simulink model "AccTarSel"  (R2018b)
settings: Solver=FixedStepDiscrete  StartTime=0.0  StopTime=inf  FixedStep=0.01  RelTol=1e-3
PostLoadFcn:
  | if any(exist('dsrtsu_mdlpostloadfcn', 'file') ~= 0), dsrtsu_mdlpostloadfcn('Execute', bdroot); end
values from neighbouring files (symbols this model uses):
  P_adtMaxBDC = 1.0    [AccTarSel.sldd]
  P_aFOCApproachIntpAcitve = -0.6    [AccTarSel.sldd]
  P_aFOCApproachIntpEnsure = -1.8    [AccTarSel.sldd]
  P_CutInEnable = 1.0    [AccTarSel.sldd]
  P_dAimMin = 4.5    [AccTarSel.sldd]
  P_dAimMinAVP = 1.5    [AccTarSel.sldd]
  P_dObjDrvOffMax = 5.0    [AccTarSel.sldd]
  P_dObjDrvOffMin = 3.0    [AccTarSel.sldd]
  P_dObjLowHystDecToStop = 4.5    [AccTarSel.sldd]
  P_dObjLowHystDecToStopAVP = 1.5    [AccTarSel.sldd]
  P_dObjUpperHystDecToStop = 5.0    [AccTarSel.sldd]
  P_dResMax = 5.0    [AccTarSel.sldd]
  P_dStandStill = 3.0    [AccTarSel.sldd]
  P_dStandStillMin = 2.0    [AccTarSel.sldd]
  P_dvarYMax4PO = 1.0    [AccTarSel.sldd]
  P_dyCutInThres = 3.6    [AccTarSel.sldd]
  P_facBDCInit = 0.7    [AccTarSel.sldd]
  P_facBDCIterCalc = 0.8    [AccTarSel.sldd]
  P_facFOCNegDiff = 0.3    [AccTarSel.sldd]
  P_facFOCPosDiff = 0.2    [AccTarSel.sldd]
  P_kapHystThres = 0.0005    [AccTarSel.sldd]
  P_PlausIntegDisable = 0.0    [AccTarSel.sldd]
  P_plausMin4PO = 0.5    [AccTarSel.sldd]
  P_probExistMin4PO = 0.8    [AccTarSel.sldd]
  P_StandObjEnable = 0.0    [AccTarSel.sldd]
  P_tAxTrackNegLower = 0.3    [AccTarSel.sldd]
  P_tAxTrackNegUpper = 0.6    [AccTarSel.sldd]
  P_tAxTrackPosLower = 1.0    [AccTarSel.sldd]
  P_tAxTrackPosUpper = 2.0    [AccTarSel.sldd]
  P_tBDCStartFilt = 0.2    [AccTarSel.sldd]
  P_tCSC = 3.5    [AccTarSel.sldd]
  P_tCurvFilt = 0.2    [AccTarSel.sldd]
  P_tCutInFilt = 0.5    [AccTarSel.sldd]
  P_tFiltAxAbsPONegFast = 0.1    [AccTarSel.sldd]
  P_tFiltAxAbsPONegSlow = 0.4    [AccTarSel.sldd]
  P_tFiltAxAbsPOPosFast = 1.2    [AccTarSel.sldd]
  P_tFiltAxAbsPOPosSlow = 2.0    [AccTarSel.sldd]
  P_tFiltAxAbsPOStand = 2.0    [AccTarSel.sldd]
  P_tFiltDAim = 0.1    [AccTarSel.sldd]
  P_tFiltDsd = 0.1    [AccTarSel.sldd]
  P_tFiltSpdLim = 3.0    [AccTarSel.sldd]
  P_tFiltVxAxPOFast = 0.15    [AccTarSel.sldd]
  P_tFiltVxAxPOSlow = 0.25    [AccTarSel.sldd]
  P_tFOCStatAccelFast = 4.0    [AccTarSel.sldd]
  P_tFOCStatAccelSlow = 3.5    [AccTarSel.sldd]
  P_tFOCStatDecelFast = 4.0    [AccTarSel.sldd]
  P_tFOCStatDecelSlow = 3.2    [AccTarSel.sldd]
  P_tMinDrvPhase = 2.0    [AccTarSel.sldd]
  P_tPredObjLeav = 1.2    [AccTarSel.sldd]
  P_tRollingFilt = 0.5    [AccTarSel.sldd]
  P_tRollingFinFilt = 1.0    [AccTarSel.sldd]
  P_tSSCNeg = 4.5    [AccTarSel.sldd]
  P_tSSCPos = 5.5    [AccTarSel.sldd]
  P_tToStop = 5.0    [AccTarSel.sldd]
  P_tToStopInBDC = 6.0    [AccTarSel.sldd]
  P_tToStopTrig = 4.0    [AccTarSel.sldd]
  P_vEgoDecToStop = 3.0    [AccTarSel.sldd]
  P_vEgoLowBDC = 4.0    [AccTarSel.sldd]
  P_vFOCNegDiff = 4.0    [AccTarSel.sldd]
  P_vFOCPosDiff = 5.0    [AccTarSel.sldd]
  P_vFOCStationaryFast = 15.0    [AccTarSel.sldd]
  P_vFOCStationarySlow = 5.0    [AccTarSel.sldd]
  P_vObjDrvOff = 0.5    [AccTarSel.sldd]
  P_vObjLowHystDecToStop = 0.5    [AccTarSel.sldd]
  P_vObjNoStop = 1.0    [AccTarSel.sldd]
  P_vObjReCalc = 1.0    [AccTarSel.sldd]
  P_vObjStop = 0.3    [AccTarSel.sldd]
  P_vObjUpperHystDecToStop = 0.8    [AccTarSel.sldd]
  P_vStandStill = 0.3    [AccTarSel.sldd]
  P_vStandStillHyst = 0.3    [AccTarSel.sldd]
  P_vyCutInThres = 0.5    [AccTarSel.sldd]
libraries: simulink x21, LPFilter x12
(part 11 of 11)

== system AccTarSel/ACC_Control/FollowObjCtrl/FollowObjValid/BrakeDistCtrl/calcA/If Action Subsystem/If Action Subsystem1 ==
  t : Inport
  aMax : Inport  Port=2
  adt2 : Inport  Port=3
  T30 : Inport  Port=4
  dRes : Inport  Port=5
  aCharactK1 : Inport  Port=6
  SYS_Info_st : Inport  Port=7
  Action Port : ActionPort  ActionType=elseif
  Add : Sum
  Add1 : Sum  Inputs=+-
  Bus Selector : BusSelector  OutputSignals=dT
  Constant : Constant
  Constant2 : Constant  Value=0  OutDataTypeStr=single
  LPFilter : LPFilter/LPFilter  SystemSampleTime=-1
      settings: SourceProductName=CustomLib
  LPFilter1 : LPFilter/LPFilter  SystemSampleTime=-1
      settings: SourceProductName=CustomLib
  Multiply : Product
  P_tRollingFilt : Constant  Value=P_tRollingFilt  OutDataTypeStr=single
  P_tRollingFinFilt : Constant  Value=P_tRollingFinFilt  OutDataTypeStr=single
  Relational Operator : RelationalOperator  Operator=>  OutDataTypeStr=boolean  RndMeth=Simplest
  Switch : Switch  Criteria=u2 > Threshold
  Out1 : Outport
  wires:
  aMax/1 -> Add/1
  t/1 -> Add1/1
  T30/1 -> Add1/2
  Add1/1 -> Multiply/1
  adt2/1 -> Multiply/2
  Multiply/1 -> Add/2
  Constant/1 -> Relational Operator/2
  dRes/1 -> Relational Operator/1
  Relational Operator/1 -> Switch/2
  Switch/1 -> Out1/1
  aCharactK1/1 -> LPFilter/4, LPFilter1/4
  SYS_Info_st/1 -> Bus Selector/1
  Bus Selector/1 -> LPFilter/2, LPFilter1/2  "<dT>"
  LPFilter/1 -> Switch/1
  P_tRollingFilt/1 -> LPFilter/3
  Constant2/1 -> LPFilter/1
  Add/1 -> LPFilter1/1
  P_tRollingFinFilt/1 -> LPFilter1/3
  LPFilter1/1 -> Switch/3

== system AccTarSel/ACC_Control/FollowObjCtrl/FollowObjValid/BrakeDistCtrl/calcA/If Action Subsystem/If Action Subsystem2 ==
  Action Port : ActionPort  ActionType=else
  Constant : Constant  Value=0  OutDataTypeStr=single
  Out1 : Outport
  wires:
  Constant/1 -> Out1/1

== system AccTarSel/ACC_Control/FollowObjCtrl/FollowObjValid/BrakeDistCtrl/calcA/If Action Subsystem/If Action Subsystem3 ==
  In1 : Inport
  Action Port : ActionPort  ActionType=then
  Out1 : Outport
  wires:
  In1/1 -> Out1/1

== system AccTarSel/ACC_Control/FollowObjCtrl/FollowObjValid/BrakeDistCtrl/calcA/If Action Subsystem/Subsystem ==
  aCharact : Inport
  a0Raw : Inport  Port=2
  tElapse : Inport  Port=3
  SYS_Info_st : Inport  Port=4
  aBDCK1 : Inport  Port=5
  Action Port : ActionPort  ActionType=else
  Bus Selector : BusSelector  OutputSignals=dT
  LPFilter : LPFilter/LPFilter  SystemSampleTime=-1
      settings: SourceProductName=CustomLib
  P_adtMaxBDC : Constant  Value=P_adtMaxBDC
  P_tBDCStartFilt : Constant  Value=P_tBDCStartFilt  OutDataTypeStr=single
  Relational Operator : RelationalOperator  Operator=<=  OutDataTypeStr=boolean  RndMeth=Simplest
  Switch : Switch  Criteria=u2 > Threshold
  Terminator : Terminator
  Out1 : Outport
  wires:
  tElapse/1 -> Relational Operator/1
  P_adtMaxBDC/1 -> Terminator/1
  a0Raw/1 -> Switch/1
  Bus Selector/1 -> LPFilter/2, Relational Operator/2  "<dT>"
  Relational Operator/1 -> Switch/2
  Switch/1 -> Out1/1
  SYS_Info_st/1 -> Bus Selector/1
  aBDCK1/1 -> LPFilter/4
  P_tBDCStartFilt/1 -> LPFilter/3
  aCharact/1 -> LPFilter/1
  LPFilter/1 -> Switch/3

== system AccTarSel/ACC_Control/FollowObjCtrl/FollowObjValid/BrakeDistCtrl/calcCriteria/calcObjStop/ObjNoStop ==
  Action Port : ActionPort  ActionType=then
  Constant2 : Constant  Value=255  OutDataTypeStr=single
  tToStop : Outport
  dToStop : Outport  Port=2
  wires:
  Constant2/1 -> dToStop/1, tToStop/1

== system AccTarSel/ACC_Control/FollowObjCtrl/FollowObjValid/BrakeDistCtrl/calcCriteria/calcObjStop/ObjStopped ==
  Action Port : ActionPort  ActionType=elseif
  Constant2 : Constant  Value=0  OutDataTypeStr=single
  tToStop : Outport
  dToStop : Outport  Port=2
  wires:
  Constant2/1 -> tToStop/1, dToStop/1

== system AccTarSel/ACC_Control/FollowObjCtrl/FollowObjValid/BrakeDistCtrl/calcCriteria/calcObjStop/ObjStopping ==
  vAbsObj : Inport
  aAbsObj : Inport  Port=2
  Action Port : ActionPort  ActionType=else
  Abs : Abs
  Abs1 : Abs
  Constant1 : Constant  Value=-0.1  OutDataTypeStr=single
  Constant2 : Constant  Value=2  OutDataTypeStr=single
  Divide1 : Product  Inputs=*/
  Divide2 : Product  Inputs=*/
  Min : MinMax  Inputs=2
  Multiply : Product
  Square : Math  Operator=square  SaturateOnIntegerOverflow=on
  tToStop : Outport
  dToStop : Outport  Port=2
  wires:
  vAbsObj/1 -> Square/1, Divide1/1
  Divide1/1 -> Abs/1
  Square/1 -> Divide2/1
  Constant2/1 -> Multiply/2
  Multiply/1 -> Divide2/2
  Divide2/1 -> Abs1/1
  Abs/1 -> tToStop/1
  Abs1/1 -> dToStop/1
  aAbsObj/1 -> Min/1
  Constant1/1 -> Min/2
  Min/1 -> Multiply/1, Divide1/2

== system AccTarSel/ACC_Control/FollowObjCtrl/FollowObjValid/BrakeDistCtrl/calcCriteria/calcObjStop/Subsystem ==
  StateK1 : Inport
  Constant2 : Constant  Value=3  OutDataTypeStr=single
  Constant3 : Constant  Value=2  OutDataTypeStr=single
  OR : Logic  Operator=OR  AllPortsSameDT=off  OutDataTypeStr=boolean
  P_tToStop : Constant  Value=P_tToStop  OutDataTypeStr=single
  P_tToStopInBDC : Constant  Value=P_tToStopInBDC  OutDataTypeStr=single
  Relational Operator : RelationalOperator  Operator===  OutDataTypeStr=boolean  RndMeth=Simplest
  Relational Operator1 : RelationalOperator  Operator===  OutDataTypeStr=boolean  RndMeth=Simplest
  Switch : Switch  Criteria=u2 > Threshold
  tStop : Outport
  wires:
  Relational Operator1/1 -> OR/2
  Relational Operator/1 -> OR/1
  OR/1 -> Switch/2
  Constant2/1 -> Relational Operator1/2
  StateK1/1 -> Relational Operator1/1, Relational Operator/1
  Constant3/1 -> Relational Operator/2
  P_tToStopInBDC/1 -> Switch/1
  P_tToStop/1 -> Switch/3
  Switch/1 -> tStop/1

== system AccTarSel/ACC_Control/FollowObjCtrl/FollowObjValid/BrakeDistCtrl/calcProfile/calc/Subsystem ==
  initCond : Inport
  Add : Sum  Inputs=+-
  Add1 : Sum  Inputs=+-
  Bus Creator : BusCreator  Inputs=8
  Bus Selector : BusSelector  OutputSignals=SmoothStopCond,a0,a0Raw
  Divide : Product  Inputs=*/
  Divide1 : Product  Inputs=*/
  Gain : Gain  Gain=-1
  Iteration : Subsystem  TreatAsAtomicUnit=on
  Profile : Outport
  wires:
  initCond/1 -> Iteration/1(initCond), Bus Selector/1
  Iteration/1(aMax) -> Bus Creator/2, Add/1, Gain/1
  Bus Selector/2 -> Bus Creator/7, Add/2  "<a0>"
  Add/1 -> Divide/1
  Iteration/3(T30) -> Bus Creator/4, Add1/2, Divide/2
  Divide/1 -> Bus Creator/5  "adt1"
  Iteration/2(T) -> Bus Creator/3, Add1/1
  Gain/1 -> Divide1/1
  Add1/1 -> Divide1/2
  Divide1/1 -> Bus Creator/6  "adt2"
  Bus Selector/1 -> Bus Creator/1  "<SmoothStopCond>"
  Bus Creator/1 -> Profile/1  "Profile"
  Bus Selector/3 -> Bus Creator/8  "<a0Raw>"

== system AccTarSel/ACC_Control/FollowObjCtrl/FollowObjValid/BrakeDistCtrl/calcProfile/calc/calcInitCondition ==
  note: a0 should be calculated by both aRef and last aCmd value
  egoInfo : Inport
  objInfo : Inport  Port=2
  dObjToStop : Inport  Port=3
  aCvK1 : Inport  Port=4
  Add : Sum  Inputs=++-
  Add1 : Sum
  Bus Selector : BusSelector  OutputSignals=aRef,vRef
  Bus Selector1 : BusSelector  OutputSignals=dx
  Constant : Constant  Value=-0.1  OutDataTypeStr=single
  Divide : Product  Inputs=*/
  Gain : Gain  Gain=-2/3
  Gain1 : Gain
  Gain2 : Gain  Gain=0.0
  Max : MinMax  Function=max  Inputs=2
  Min : MinMax  Inputs=2
  Multiply : Product
  Multiply1 : Product
  P_dStandStill : Constant  Value=P_dStandStill  OutDataTypeStr=single
  P_dStandStillMin : Constant  Value=P_dStandStillMin  OutDataTypeStr=single
  P_facBDCInit : Constant  Value=P_facBDCInit  OutDataTypeStr=single
  Square : Math  Operator=square  SaturateOnIntegerOverflow=on
  a0 : Outport
  aThres : Outport  Port=2
  v0 : Outport  Port=3
  v30 : Outport  Port=4
  dAimBDC : Outport  Port=5
  d30 : Outport  Port=6
  wires:
  egoInfo/1 -> Bus Selector/1
  Bus Selector/2 -> Multiply/1, v0/1, Square/1  "<vRef>"
  objInfo/1 -> Bus Selector1/1
  dObjToStop/1 -> Add/2
  Bus Selector1/1 -> Add/1  "<dx>"
  P_dStandStill/1 -> Add/3
  Add/1 -> Max/1
  P_dStandStillMin/1 -> Max/2
  Max/1 -> Divide/2, Multiply1/1, dAimBDC/1  "dAimBDC"
  Square/1 -> Divide/1
  Divide/1 -> Gain/1
  Gain/1 -> aThres/1
  Multiply/1 -> v30/1
  P_facBDCInit/1 -> Multiply1/2, Multiply/2
  Multiply1/1 -> d30/1
  aCvK1/1 -> Gain1/1
  Bus Selector/1 -> Gain2/1  "<aRef>"
  Gain1/1 -> Add1/1
  Gain2/1 -> Add1/2
  Add1/1 -> Min/2
  Constant/1 -> Min/1
  Min/1 -> a0/1

== system AccTarSel/ACC_Target_Selection/Subsystem/ValidObjCalc/CutInCalc/Subsystem/Subsystem/If Action Subsystem ==
  dy : Inport
  vy : Inport  Port=2
  Action Port : ActionPort  ActionType=then
  1-D Lookup Table : Lookup_n-D  NumberOfTableDimensions=1  LookupTableObject=''  BreakpointsForDimension1=[0.5,1.5]  BreakpointsForDimension1FirstPoint=10  BreakpointsForDimension2FirstPoint=10  BreakpointsForDimension1Spacing=12  BreakpointsForDimension2Spacing=12  IndexSearchMethod=Linear search  Table=[0,1.5]  ExtrapMethod=Clip  InternalRulePriority=Speed  RndMeth=Simplest  InputSameDT=on
  1-D Lookup Table1 : Lookup_n-D  NumberOfTableDimensions=1  LookupTableObject=''  BreakpointsForDimension1=[1,1.8]  BreakpointsForDimension1FirstPoint=10  BreakpointsForDimension2FirstPoint=10  BreakpointsForDimension1Spacing=12  BreakpointsForDimension2Spacing=12  IndexSearchMethod=Linear search  Table=[1,0]  ExtrapMethod=Clip  InternalRulePriority=Speed  RndMeth=Simplest  InputSameDT=on
  Abs : Abs
  Abs1 : Abs
  Add : Sum
  Constant : Constant  Value=0  OutDataTypeStr=single
  Max : MinMax  Function=max  Inputs=2
  Max1 : MinMax  Inputs=2
  Multiply : Product
  Switch : Switch  Criteria=u2 > Threshold
  Out1 : Outport
  Out2 : Outport  Port=2
  wires:
  vy/1 -> Multiply/1, Abs1/1
  1-D Lookup Table/1 -> Multiply/2  "tPred"
  dy/1 -> Switch/2, Add/1
  Multiply/1 -> Add/2
  Add/1 -> Max1/2, Max/1
  Constant/1 -> Max1/1, Max/2
  Switch/1 -> Out2/1, Abs/1  "dyPred"
  1-D Lookup Table1/1 -> Out1/1
  Abs/1 -> 1-D Lookup Table1/1
  Abs1/1 -> 1-D Lookup Table/1
  Max/1 -> Switch/1
  Max1/1 -> Switch/3

== system AccTarSel/ACC_Target_Selection/Subsystem/ValidObjCalc/CutInCalc/Subsystem/Subsystem/If Action Subsystem1 ==
  dy : Inport
  Action Port : ActionPort  ActionType=else
  Constant : Constant  Value=0  OutDataTypeStr=single
  Out1 : Outport
  Out2 : Outport  Port=2
  wires:
  Constant/1 -> Out1/1
  dy/1 -> Out2/1

== system AccTarSel/ACC_Control/FollowObjCtrl/FollowObjValid/BrakeDistCtrl/calcProfile/calc/Subsystem/Iteration ==
  initCond : Inport
  Add : Sum  Inputs=+-
  Add1 : Sum
  Add2 : Sum
  Add3 : Sum  Inputs=+++
  Bus Selector : BusSelector  OutputSignals=dAimBDC,d30,v30,a0,v0
  Constant : Constant  OutDataTypeStr=int32
  Divide : Product  Inputs=*/
  Divide1 : Product  Inputs=*/
  For Iterator : ForIterator  IterationLimit=10
  Gain : Gain  Gain=0.7
  Gain1 : Gain  Gain=3
  Gain2 : Gain  Gain=0.7
  Gain3 : Gain  Gain=-2
  Gain4 : Gain  Gain=0.3
  Gain5 : Gain  Gain=0.5
  Gain6 : Gain  Gain=1/3
  Gain7 : Gain  Gain=1/6
  Gain8 : Gain  Gain=0.3
  Memory{,1..3} (4 alike) : Memory  InheritSampleTime=on
  Multiply{,1..3} (4 alike) : Product
  Relational Operator : RelationalOperator  Operator===  OutDataTypeStr=boolean  RndMeth=Simplest
  Square : Math  Operator=square  SaturateOnIntegerOverflow=on
  calcD30 : Subsystem
  calcV30 : Subsystem
  aMax : Outport
  T : Outport  Port=2
  T30 : Outport  Port=3
  wires:
  initCond/1 -> Bus Selector/1
  Bus Selector/1 -> Add/1  "<dAimBDC>"
  calcD30/1(d30) -> Add/2, Memory2/1  "d30"
  calcV30/1(v30) -> Memory3/1, Gain/1, Gain3/1  "v30"
  Add/1 -> Divide/1
  Gain/1 -> Divide/2
  Divide/1 -> Gain1/1
  Gain1/1 -> Gain8/1, T/1, Gain4/1, Gain2/1  "T"
  Gain3/1 -> Divide1/1
  Gain2/1 -> Divide1/2  "0.7T"
  Divide1/1 -> aMax/1, Multiply3/1, Add2/1  "aMax"
  Gain4/1 -> Multiply1/1, Square/1, Multiply/2  "0.3T"
  Bus Selector/4 -> Multiply2/1, Add2/2  "<a0>"
  Multiply/1 -> Gain5/1
  Gain5/1 -> Add1/1
  Bus Selector/5 -> Multiply1/2, Add1/2  "<v0>"
  Add2/1 -> Multiply/1
  Add1/1 -> Memory1/1  "v30new"
  Square/1 -> Multiply3/2, Multiply2/2
  Multiply2/1 -> Gain6/1
  Multiply3/1 -> Gain7/1
  Gain6/1 -> Add3/1
  Gain7/1 -> Add3/2
  Multiply1/1 -> Add3/3
  Add3/1 -> Memory/1  "d30new"
  For Iterator/1 -> Relational Operator/1
  Constant/1 -> Relational Operator/2
  Relational Operator/1 -> calcD30/2(first_Iteration), calcV30/2(first_Iteration)
  Bus Selector/2 -> calcD30/1(d30Init)  "<d30>"
  Memory/1 -> calcD30/3(d30New)
  Memory1/1 -> calcV30/3(v30new)
  Bus Selector/3 -> calcV30/1(v30Init)  "<v30>"
  Gain8/1 -> T30/1  "T30"
  Memory2/1 -> calcD30/4(d30Old)
  Memory3/1 -> calcV30/4(v30Old)

== system AccTarSel/ACC_Control/FollowObjCtrl/FollowObjValid/BrakeDistCtrl/calcProfile/calc/Subsystem/Iteration/calcD30 ==
  d30Init : Inport
  first_Iteration : Inport  Port=2
  d30New : Inport  Port=3
  d30Old : Inport  Port=4
  Add : Sum  Inputs=+-
  Add1 : Sum
  Constant1 : Constant  OutDataTypeStr=single
  Multiply : Product
  Multiply1 : Product
  P_facBDCIterCalc : Constant  Value=P_facBDCIterCalc
  Switch : Switch  Criteria=u2 > Threshold
  d30 : Outport
  wires:
  d30Init/1 -> Switch/1
  first_Iteration/1 -> Switch/2
  Switch/1 -> d30/1
  P_facBDCIterCalc/1 -> Multiply/2, Add/2
  Constant1/1 -> Add/1
  Add/1 -> Multiply1/1
  d30New/1 -> Multiply1/2
  Multiply1/1 -> Add1/2
  Multiply/1 -> Add1/1
  Add1/1 -> Switch/3
  d30Old/1 -> Multiply/1

== system AccTarSel/ACC_Control/FollowObjCtrl/FollowObjValid/BrakeDistCtrl/calcProfile/calc/Subsystem/Iteration/calcV30 ==
  v30Init : Inport
  first_Iteration : Inport  Port=2
  v30new : Inport  Port=3
  v30Old : Inport  Port=4
  Add : Sum  Inputs=+-
  Add1 : Sum
  Constant1 : Constant  OutDataTypeStr=single
  Multiply : Product
  Multiply1 : Product
  P_facBDCIterCalc : Constant  Value=P_facBDCIterCalc
  Switch : Switch  Criteria=u2 > Threshold
  v30 : Outport
  wires:
  Add1/1 -> Switch/3
  Multiply/1 -> Add1/1
  Multiply1/1 -> Add1/2
  v30new/1 -> Multiply1/2
  Add/1 -> Multiply1/1
  Constant1/1 -> Add/1
  P_facBDCIterCalc/1 -> Add/2, Multiply/2
  Switch/1 -> v30/1
  first_Iteration/1 -> Switch/2
  v30Init/1 -> Switch/1
  v30Old/1 -> Multiply/1

== stateflow chart AccTarSel/ACC_Control/FollowObjCtrl/FollowObjValid/BrakeDistCtrl/BDC_State_Machine ==
  state PASSIVE
    en:
    BDC_State = 0;
    tElapse = 0;
  state ACTIVE
    en:
    BDC_State = 2;
    tElapse = tElapse + SYS_Info_st.dT;
    du:
    tElapse = tElapse + SYS_Info_st.dT;
  state RECALC
    en:
    BDC_State = 3;
    tElapse = SYS_Info_st.dT;
  state CALC
    en:
    BDC_State = 1;
    tElapse = 0;
  (default) -> PASSIVE
  ACTIVE -> PASSIVE [order 1] : [~(ObjToStop == 1&&egoLowSpd == 1)]
  CALC -> PASSIVE [order 1] : [~(ObjToStop == 1&&egoLowSpd == 1)]
  PASSIVE -> CALC : [ObjToStop == 1&&egoLowSpd == 1]
  ACTIVE -> RECALC [order 2] : [ProfileReCalc == 1]
  RECALC -> ACTIVE [order 1] : [ObjToStopTrig == 1 || PreStop == 1]
  RECALC -> CALC [order 2] : [~(ObjToStopTrig == 1 || PreStop == 1)]
  CALC -> ACTIVE [order 2] : [ObjToStopTrig == 1 || PreStop == 1]
  data: ObjToStop input; ObjToStopTrig input; egoLowSpd input; PreStop input boolean; ProfileReCalc input; BDC_State output single; tElapse output single; SYS_Info_st input

== stateflow chart AccTarSel/ACC_State_Machine1 ==
  note: MainState
      | 0	OFF
      | 1	PASSIVE
      | 2	ACTIVE_Drive
      | 3	ACTIVE_Standstill
      | 4	OVERRIDE
  state OFF
    en:
    AST_Info_st.MainState = 0;
    AST_Info_st.tMinInDrv = 0;
    AST_Info_st.vSet = 0;
  state OVERRIDE
    en:
    AST_Info_st.MainState = 4;
    AST_Info_st.tMinInDrv = 0;
  state PASSIVE
    en:
    AST_Info_st.MainState = 1;
    AST_Info_st.tMinInDrv = 0;
  state ACTIVE
    en:
    if ((NET_DrvAction_st.ACC_SetSw == 1)&&(NET_DrvAction_st.ACC_SetSwK1 == 0))
    AST_Info_st.vSet = round(VSI_VehState_st.vRef*1.05*3.6)/1.05/3.6;
    end
    AST_Info_st.vSet = min(AST_Info_st.vSet, (100/1.05)/3.6);
    AST_Info_st.vSet = max(AST_Info_st.vSet, (30/1.05)/3.6);
    du:
    if ((NET_DrvAction_st.ACC_SpdIncSw == 1)&&(NET_DrvAction_st.ACC_SpdIncSwK1 == 0))
    AST_Info_st.vSet = AST_Info_st.vSet + (5 - mod(round(AST_Info_st.vSet*1.05*3.6),5))/1.05/3.6;
    else if ((NET_DrvAction_st.ACC_SpdDecSw == 1)&&(NET_DrvAction_st.ACC_SpdDecSwK1 == 0))
    AST_Info_st.vSet = AST_Info_st.vSet + (mod(5 - mod(round(AST_Info_st.vSet*1.05*3.6),5),5))/1.05/3.6 - 5/1.05/3.6;
    end
    end
    if (ZOP_Enable == 1)
    if (vSet_HMI.vSetAccSpd >= 60)
    AST_Info_st.vSet = vSet_HMI.vSetAccSpd/1.05/3.6;
    end
    else
    if (vSet_HMI.vSetAccSpd >= 30)
    AST_Info_st.vSet = vSet_HMI.vSetAccSpd/1.05/3.6;
    end
    end
    AST_Info_st.vSet = min(AST_Info_st.vSet, (100/1.05)/3.6);
    AST_Info_st.vSet = max(AST_Info_st.vSet, (30/1.05)/3.6);
    state Drive
      en:
      AST_Info_st.MainState = 2;
      du:
      if(VSI_VehState_st.vRef > P_vStandStillHyst)
      if(AST_Info_st.tMinInDrv > SYS_Info_st.dT)
      AST_Info_st.tMinInDrv = AST_Info_st.tMinInDrv - SYS_Info_st.dT;
      else
      AST_Info_st.tMinInDrv = 0;
      end
      end
    state Standstill
      en:
      AST_Info_st.MainState = 3;
      AST_Info_st.tMinInDrv = P_tMinDrvPhase;
    (default) -> Drive
    Drive -> Standstill : [VSI_VehState_st.vRef < P_vStandStill...
        | &&AST_Info_st.tMinInDrv == 0]
    Standstill -> Drive : [DrvOffEnable == 1]
  (default) -> OFF
  OVERRIDE -> OFF [order 3] : [NET_DrvAction_st.ACC_MainSw == 0]
  ACTIVE -> OFF [order 3] : [NET_DrvAction_st.ACC_MainSw == 0]
  OVERRIDE -> PASSIVE [order 2] : [NET_DrvAction_st.ACC_CancelSw == 1||NET_DrvAction_st.BrakePedalApply == 1||NET_DrvAction_st.GearLever < 3]
  ACTIVE -> OVERRIDE [order 1] : [NET_DrvAction_st.DrvOverride == 1]
  OVERRIDE -> ACTIVE [order 1] : [NET_DrvAction_st.DrvOverride == 0]
  OFF -> PASSIVE : [NET_DrvAction_st.ACC_MainSw == 1]
  PASSIVE -> OFF [order 2] : [NET_DrvAction_st.ACC_MainSw == 0]
  PASSIVE -> ACTIVE [order 1] : [(NET_DrvAction_st.ACC_SetSw == 1||(NET_DrvAction_st.ACC_ResSw == 1&&AST_Info_st.vSet ~= 0))&&NET_DrvAction_st.BrakePedalApply == 0&&NET_DrvAction_st.GearLever >= 3]
  ACTIVE -> PASSIVE [order 2] : [NET_DrvAction_st.ACC_CancelSw == 1||NET_DrvAction_st.BrakePedalApply == 1||NET_DrvAction_st.GearLever < 3]
  data: NET_DrvAction_st input; AST_Info_st output Bus: AST_INFO_ST; VSI_VehState_st input; DrvOffEnable input; SYS_Info_st input; P_tMinDrvPhase input; P_vStandStill input; P_vStandStillHyst input; vSet_HMI input Bus: ACC_HMI_REQ; ZOP_Enable input boolean
